simulink model "part1_model_6422780500"  (R2023a)
settings: Solver=FixedStepAuto  StartTime=0.0  StopTime=5  FixedStep=1e-4  RelTol=1e-3
InitFcn:
  | A1 = 0.09;
  | A2 = 0.09;
  | R1 = 0.5;
  | R2 = 1.0;
settings Model: Creator=LabCom  LastModifiedBy=LabCom

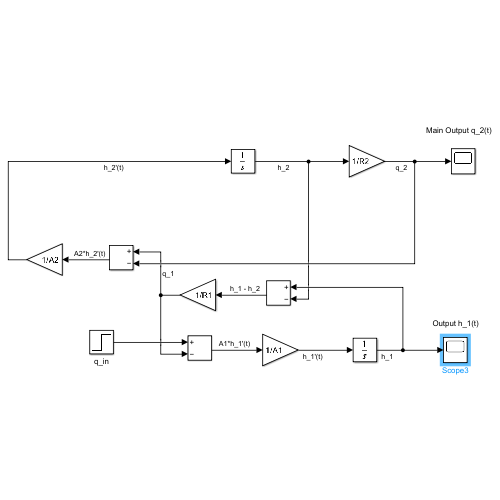
[thumbnail: Simulink's stored preview of the top-level diagram]
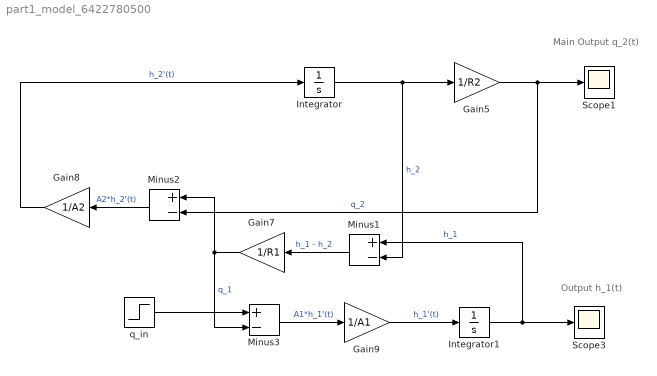
== system part1_model_6422780500 ==
  note: Main Output q_2(t)
  note: Output h_1(t)
  Gain5 : Gain  Gain=1/R2
  Gain7 : Gain  Gain=1/R1
  Gain8 : Gain  Gain=1/A2
  Gain9 : Gain  Gain=1/A1
  Integrator : Integrator
  Integrator1 : Integrator  InitialCondition=1
  Minus1 : Sum  Inputs=+-
  Minus2 : Sum  Inputs=+-
  Minus3 : Sum  Inputs=+-
  Scope1 : Scope
  Scope3 : Scope
  q_in : Step  Time=0  SampleTime=0
  wires:
  Integrator/1 -> Minus1/2, Gain5/1  "h_2"
  Gain5/1 -> Minus2/2, Scope1/1  "q_2"
  Minus1/1 -> Gain7/1  "h_1 - h_2"
  Gain7/1 -> Minus2/1, Minus3/2  "q_1"
  Minus2/1 -> Gain8/1  "A2*h_2'(t)"
  Gain8/1 -> Integrator/1  "h_2'(t)"
  q_in/1 -> Minus3/1
  Minus3/1 -> Gain9/1  "A1*h_1'(t)"
  Gain9/1 -> Integrator1/1  "h_1'(t)"
  Integrator1/1 -> Scope3/1, Minus1/1  "h_1"
